simulink model "Simulacao_sem_pertubacao"  (R2016b)
settings: Solver=VariableStepAuto  StartTime=0.0  StopTime=40.0  RelTol=1e-3
InitFcn:
  | clc; clear;
  | main
values from neighbouring files (symbols this model uses):
  Tof = Tif + Tbarra    (= 85)    [main.m]
libraries: cstblocks x2
settings Model: Creator=tiago_lobao  LastModifiedBy=tiago_lobao

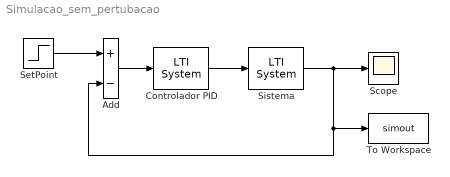
== system Simulacao_sem_pertubacao ==
  Add : Sum  Inputs=+-
  "Controlador PID " : cstblocks/LTI System  sys=C  IC=[]
  Scope : Scope
  SetPoint : Step  After=Tof  SampleTime=0
  Sistema : cstblocks/LTI System  sys=G  IC=[]
  To Workspace : ToWorkspace  VariableName=simout  SaveFormat=Timeseries  SampleTime=-1
  wires:
  Add/1 -> "Controlador PID "/1
  Sistema/1 -> Add/2, To Workspace/1, Scope/1
  SetPoint/1 -> Add/1
  "Controlador PID "/1 -> Sistema/1
